simulink model "WK1L1_sim"  (R2018b)
settings: Solver=VariableStepAuto  StartTime=0.0  StopTime=10.0  RelTol=1e-3
values from neighbouring files (symbols this model uses):
  f1 = 50    [WK1L1.m]
  L_l1 = 1e-3    (= 0.001)    [WK1L1.m]
  L_l2d = 2e-3    (= 0.002)    [WK1L1.m]
  L_m1 = 20e-3    (= 0.02)    [WK1L1.m]
  r1 = 1    [WK1L1.m]
  r2d = 2    [WK1L1.m]
  r_ld = 50    [WK1L1.m]
  v1 = 200    [WK1L1.m]
libraries: simulink x1
settings Model: Creator=Job  LastModifiedBy=Job

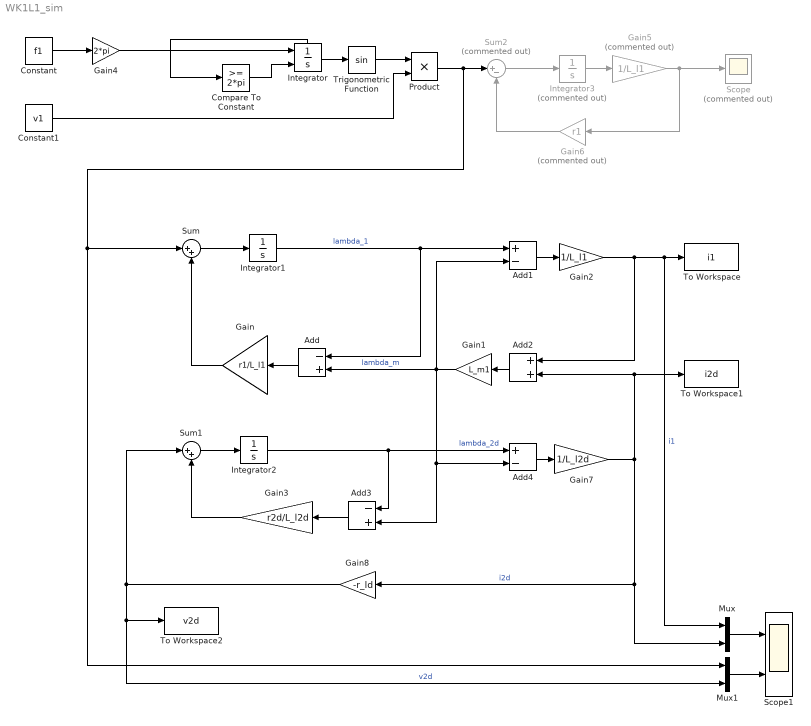
== system WK1L1_sim ==
  Add : Sum  Inputs=-+
  Add1 : Sum  Inputs=+-
  Add2 : Sum
  Add3 : Sum  Inputs=-+
  Add4 : Sum  Inputs=+-
  Compare To Constant : simulink/Logic and Bit Operations/Compare To Constant  relop=>=  const=2*pi  OutDataTypeStr=boolean
  Constant : Constant  Value=f1
  Constant1 : Constant  Value=v1
  Gain : Gain  Gain=r1/L_l1
  Gain1 : Gain  Gain=L_m1
  Gain2 : Gain  Gain=1/L_l1
  Gain3 : Gain  Gain=r2d/L_l2d
  Gain4 : Gain  Gain=2*pi
  Gain5 : Gain  Commented=on  Gain=1/L_l1
  Gain6 : Gain  Commented=on  Gain=r1
  Gain7 : Gain  Gain=1/L_l2d
  Gain8 : Gain  Gain=-r_ld
  Integrator : Integrator  ExternalReset=rising  ShowStatePort=on
  Integrator1 : Integrator
  Integrator2 : Integrator
  Integrator3 : Integrator  Commented=on
  Mux : Mux  Inputs=2
  Mux1 : Mux  Inputs=2
  Product : Product
  Scope : Scope  Commented=on
  Scope1 : Scope  NumInputPorts=2
  Sum : Sum  Inputs=|++
  Sum1 : Sum  Inputs=|++
  Sum2 : Sum  Commented=on  Inputs=|+-
  To Workspace : ToWorkspace  VariableName=i1  SaveFormat=Timeseries  SampleTime=-1
  To Workspace1 : ToWorkspace  VariableName=i2d  SaveFormat=Timeseries  SampleTime=-1
  To Workspace2 : ToWorkspace  VariableName=v2d  SaveFormat=Timeseries  SampleTime=-1
  Trigonometric Function : Trigonometry
  wires:
  Constant/1 -> Gain4/1
  Integrator/1 -> Trigonometric Function/1
  Compare To Constant/1 -> Integrator/2
  Integrator/State -> Compare To Constant/1
  Trigonometric Function/1 -> Product/1
  Constant1/1 -> Product/2
  Integrator1/1 -> Add/1, Add1/1  "lambda_1"
  Sum/1 -> Integrator1/1
  Product/1 -> Sum/1, Mux1/1, Sum2/1
  Gain1/1 -> Add4/2, Add3/2, Add1/2, Add/2  "lambda_m"
  Add/1 -> Gain/1
  Gain/1 -> Sum/2
  Add2/1 -> Gain1/1
  Gain2/1 -> Add2/1, Mux/1, To Workspace/1  "i1"
  Gain7/1 -> Mux/2, Gain8/1, Add2/2, To Workspace1/1  "i2d"
  Add1/1 -> Gain2/1
  Sum1/1 -> Integrator2/1
  Gain8/1 -> Sum1/1, Mux1/2, To Workspace2/1  "v2d"
  Gain3/1 -> Sum1/2
  Add3/1 -> Gain3/1
  Integrator2/1 -> Add4/1, Add3/1  "lambda_2d"
  Gain4/1 -> Integrator/1
  Sum2/1 -> Integrator3/1
  Integrator3/1 -> Gain5/1
  Gain6/1 -> Sum2/2
  Gain5/1 -> Scope/1, Gain6/1
  Add4/1 -> Gain7/1
  Mux/1 -> Scope1/1
  Mux1/1 -> Scope1/2
